simulink model "automodel_discreet"  (R2017b)
settings: Solver=ode4  StartTime=0.0  StopTime=200  FixedStep=0.01  RelTol=1e-3
undefined symbols (not defined in the file): DiscIntNeverNeededParam
settings Model: Creator=Kris  LastModifiedBy=Kris
settings OptimizationCC: DefaultParameterBehavior=Inlined  PassReuseOutputArgsAs=Individual arguments
settings DebuggingCC: AlgebraicLoopMsg=none  ParameterTunabilityLossMsg=error
settings SFSimCC: MATLABDynamicMemAlloc=off
settings RTWCC: SystemTargetFile=ert.tlc  TemplateMakefile=ert_default_tmf  GenerateReport=on  IncludeHyperlinkInReport=on  LaunchReport=on  GenerateTraceInfo=on  GenerateTraceReport=on  GenerateTraceReportSl=on  GenerateTraceReportSf=on  GenerateTraceReportEml=on
settings CodeAppCC: ForceParamTrailComments=on  IgnoreCustomStorageClasses=off  OperatorAnnotations=on  SimulinkDataObjDesc=on  SFDataObjDesc=on  InsertBlockDesc=on
settings ERTTargetCC: TargetLangStandard=C99 (ISO)  GenerateSampleERTMain=on  InlinedParameterPlacement=NonHierarchical  ERTCustomFileTemplate=example_file_process.tlc

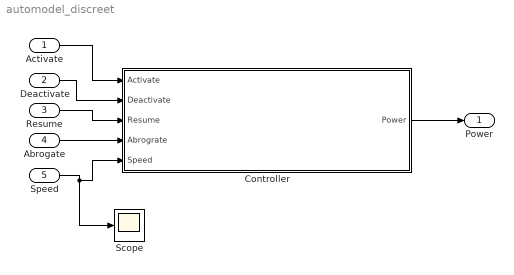
== system automodel_discreet ==
  Activate : Inport
  Deactivate : Inport  Port=2
  Resume : Inport  Port=3
  Abrogate : Inport  Port=4
  Speed : Inport  Port=5
  "Controller " : Subsystem
  Scope : Scope
  Power : Outport
  wires:
  "Controller "/1(Power) -> Power/1
  Activate/1 -> "Controller "/1(Activate)
  Deactivate/1 -> "Controller "/2(Deactivate)
  Resume/1 -> "Controller "/3(Resume)
  Abrogate/1 -> "Controller "/4(Abrograte)
  Speed/1 -> Scope/1, "Controller "/5(Speed)

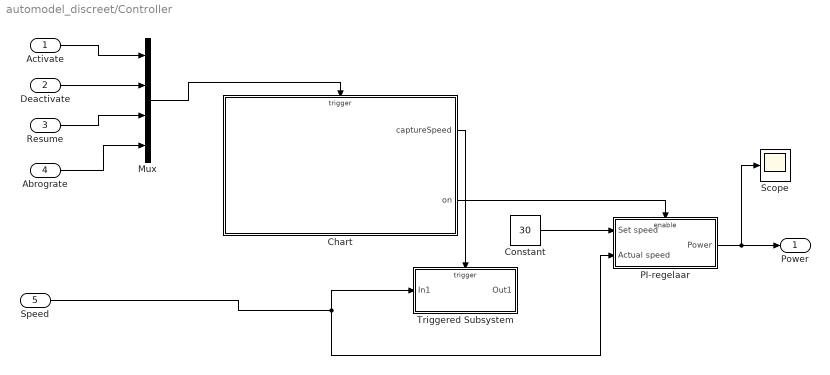
== system automodel_discreet/Controller  ==
  Activate : Inport
  Deactivate : Inport  Port=2
  Resume : Inport  Port=3
  Abrograte : Inport  Port=4
  Speed : Inport  Port=5
  Chart : Stateflow chart  TreatAsAtomicUnit=on
  Constant : Constant  Value=30
  Mux : Mux
  "PI-regelaar " : Subsystem
  Scope : Scope
  Triggered Subsystem : Subsystem  TreatAsAtomicUnit=on
  Power : Outport
  wires:
  Chart/2(on) -> "PI-regelaar "/Enable
  "PI-regelaar "/1(Power) -> Scope/1, Power/1
  Deactivate/1 -> Mux/2
  Activate/1 -> Mux/1
  Resume/1 -> Mux/3
  Abrograte/1 -> Mux/4
  Mux/1 -> Chart/Trigger
  Chart/1(captureSpeed) -> Triggered Subsystem/Trigger
  Speed/1 -> "PI-regelaar "/2(Actual speed), Triggered Subsystem/1(In1)
  Constant/1 -> "PI-regelaar "/1(Set speed)

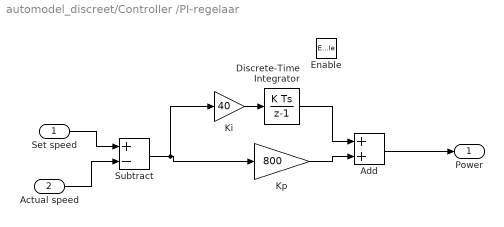
== system automodel_discreet/Controller /PI-regelaar  ==
  Set speed : Inport
  Actual speed : Inport  Port=2
  Enable : EnablePort
  Add : Sum
  Discrete-Time Integrator : DiscreteIntegrator  InitialConditionSetting=State (most efficient)  SampleTime=-1  ICPrevOutput=DiscIntNeverNeededParam  ICPrevScaledInput=DiscIntNeverNeededParam
  Ki : Gain  Gain=40
  Kp : Gain  Gain=800
  Subtract : Sum  Inputs=+-
  Power : Outport
  wires:
  Kp/1 -> Add/2
  Actual speed/1 -> Subtract/2
  Subtract/1 -> Ki/1, Kp/1
  Set speed/1 -> Subtract/1
  Add/1 -> Power/1
  Ki/1 -> Discrete-Time Integrator/1
  Discrete-Time Integrator/1 -> Add/1

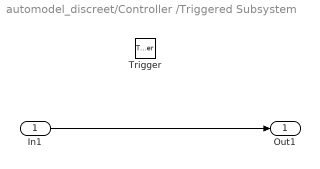
== system automodel_discreet/Controller /Triggered Subsystem ==
  In1 : Inport
  Trigger : TriggerPort  VariantControl=Variant
  Out1 : Outport
  wires:
  In1/1 -> Out1/1

== stateflow chart automodel_discreet/Controller /Chart ==
  settings: executeAtInitialization=1
  state StateOff
    entry: on = 0;
    captureSpeed = 0;
  state StateOn
    entry: on = 1
    captureSpeed =1
  state stateSuspended
    entry: on = 0
    captureSpeed = 1;
  (default) -> StateOff
  StateOn -> StateOff [order 2] : deactivate
  stateSuspended -> StateOff [order 2] : deactivate
  StateOff -> StateOn : activate
  StateOn -> stateSuspended [order 1] : abrogate
  stateSuspended -> StateOn [order 1] : resume
  data: captureSpeed output; on output
  events: activate input RISING_EDGE_EVENT; deactivate input RISING_EDGE_EVENT; resume input RISING_EDGE_EVENT; abrogate input RISING_EDGE_EVENT
